simulink model "DELAY_AND_ADD_BLOCK"  (R2022b)
settings: Solver=FixedStepDiscrete  StartTime=0.0  StopTime=10.0  RelTol=1e-3
settings Model: DataTypeOverride=Off  Creator=saran  LastModifiedBy=saran
settings SolverCC: AlgebraicLoopSolver=TrustRegion
settings DataIOCC: LimitDataPoints=on  SaveOutput=off  SaveTime=off
settings OptimizationCC: BlockReduction=off  ConditionallyExecuteInputs=off  DefaultParameterBehavior=Inlined  DefaultUnderspecifiedDataType=single  LifeSpan=inf
settings DebuggingCC: AlgebraicLoopMsg=error  SingleTaskRateTransMsg=error  UnconnectedInputMsg=warning  UnconnectedOutputMsg=warning  UnconnectedLineMsg=warning  AllowSymbolicDim=off  StrictBusMsg=ErrorOnBusTreatedAsVector  SFUnexpectedBacktrackingDiag=warning  SFNoUnconditionalDefaultTransitionDiag=warning  SFExecutionAtInitializationDiag=none  SFMachineParentedDataDiag=warning  ArithmeticOperatorsInVariantConditions=warning
settings HardwareCC: ProdBitPerPointer=32  ProdBitPerSizeT=32  ProdBitPerPtrDiffT=32  ProdLargestAtomicFloat=None  ProdIntDivRoundTo=Undefined  ProdEndianess=Unspecified  ProdWordSize=32  ProdHWDeviceType=ASIC/FPGA->ASIC/FPGA  ProdEqTarget=off
settings ModelReferenceCC: EnableRefExpFcnMdlSchedulingChecks=on
settings SFSimCC: SimUseLocalCustomCode=off  CustomCodeUndefinedFunction=UseInterfaceOnly
settings RTWCC: RTWUseLocalCustomCode=off
settings CodeAppCC: StateflowObjectComments=on
settings GRTTargetCC: TargetLangStandard=C89/C90 (ANSI)
settings ConfigComp: CovScope=ReferencedModels  CovMetricSettings=dw  CovSaveCumulativeToWorkspaceVar=on  CovSaveSingleToWorkspaceVar=on  CovExternalEMLEnable=off  CovSFcnEnable=off

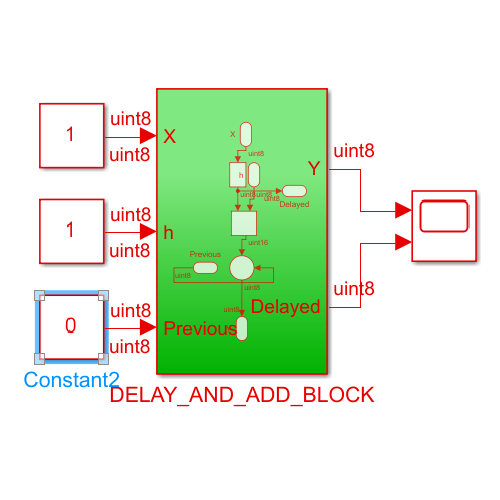
[thumbnail: Simulink's stored preview of the top-level diagram]
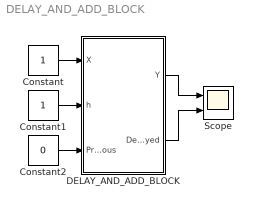
== system DELAY_AND_ADD_BLOCK ==
  Constant : Constant  OutDataTypeStr=uint8  SampleTime=1
  Constant1 : Constant  OutDataTypeStr=uint8  SampleTime=1
  Constant2 : Constant  Value=0  OutDataTypeStr=uint8  SampleTime=1
  DELAY_AND_ADD_BLOCK : Subsystem
  Scope : Scope  NumInputPorts=2
  wires:
  Constant2/1 -> DELAY_AND_ADD_BLOCK/3(Previous)
  Constant1/1 -> DELAY_AND_ADD_BLOCK/2(h)
  Constant/1 -> DELAY_AND_ADD_BLOCK/1(X)
  DELAY_AND_ADD_BLOCK/1(Y) -> Scope/1
  DELAY_AND_ADD_BLOCK/2(Delayed) -> Scope/2

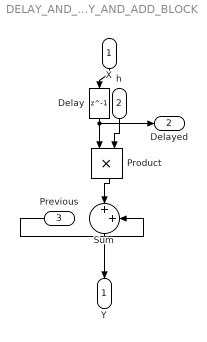
== system DELAY_AND_ADD_BLOCK/DELAY_AND_ADD_BLOCK ==
  X : Inport  OutDataTypeStr=uint8  SampleTime=1
  h : Inport  Port=2  OutDataTypeStr=uint8  SampleTime=1
  Previous : Inport  Port=3  OutDataTypeStr=uint8  SampleTime=1
  Delay : Delay  DelayLength=1  InitialCondition=0
  Product : Product
  Sum : Sum  Inputs=|++  AccumDataTypeStr=uint8  OutDataTypeStr=uint8  LockScale=on
  Y : Outport  OutDataTypeStr=uint8  SampleTime=1  VectorParamsAs1DForOutWhenUnconnected=off
  Delayed : Outport  Port=2  OutDataTypeStr=uint8  SampleTime=1  VectorParamsAs1DForOutWhenUnconnected=off
  wires:
  h/1 -> Product/2
  X/1 -> Delay/1
  Delay/1 -> Product/1, Delayed/1
  Product/1 -> Sum/1
  Previous/1 -> Sum/2
  Sum/1 -> Y/1
